simulink model "Sistema_3 (1)"  (R2025b)
settings: Solver=ode23t  StartTime=0.0  StopTime=10.0  RelTol=1e-3
libraries: fl_lib x21, nesl_utility x9, slpidlib x2
settings DataIOCC: ReturnWorkspaceOutputs=off  TimeSaveName=t
settings DebuggingCC: AlgebraicLoopMsg=none  ArtificialAlgebraicLoopMsg=none  MaxConsecutiveZCsMsg=none

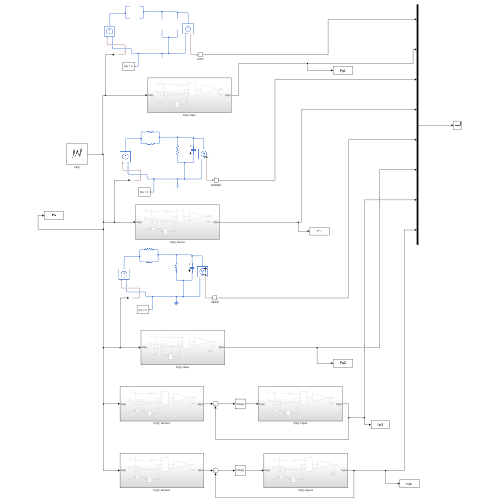
[thumbnail: Simulink's stored preview of the top-level diagram]
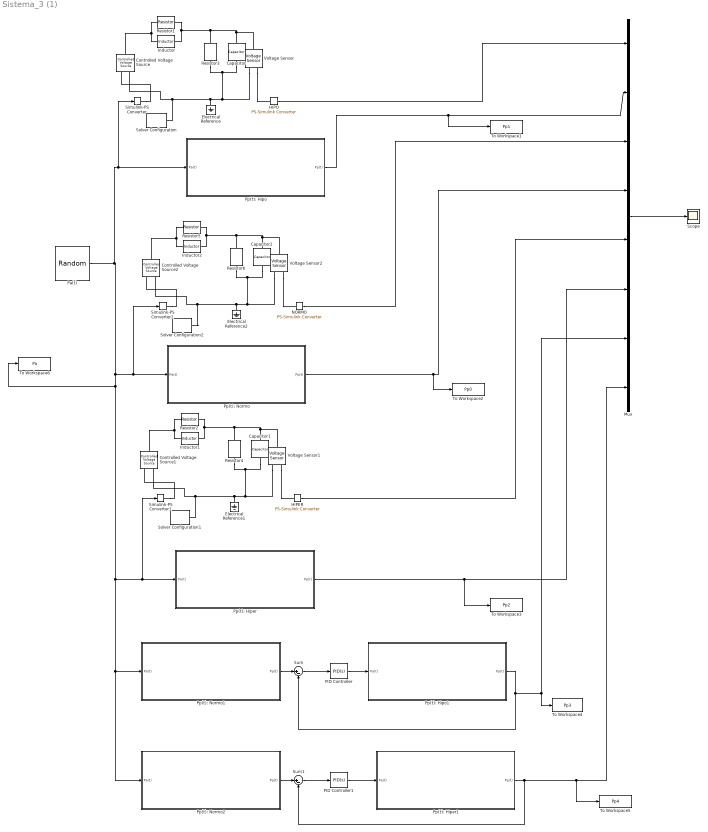
== system Sistema_3 (1) ==
  Capacitor : fl_lib/Electrical/Electrical Elements/Capacitor  c=0.005 F  r=1e-6 Ohm  g=0 1/Ohm  i_specify=off  i_priority=None  i=0 A  i_nominal_specify=off  i_nominal_value=1  i_nominal_unit=A  v_specify=off  v_priority=None  v=0 V  v_nominal_specify=off  v_nominal_value=1  v_nominal_unit=V  vc_specify=off  vc_priority=High  vc=0 V  vc_nominal_specify=off  vc_nominal_value=1  vc_nominal_unit=V
  Capacitor1 : fl_lib/Electrical/Electrical Elements/Capacitor  c=2.500 F  r=1e-6 Ohm  g=0 1/Ohm  i_specify=off  i_priority=None  i=0 A  i_nominal_specify=off  i_nominal_value=1  i_nominal_unit=A  v_specify=off  v_priority=None  v=0 V  v_nominal_specify=off  v_nominal_value=1  v_nominal_unit=V  vc_specify=off  vc_priority=High  vc=0 V  vc_nominal_specify=off  vc_nominal_value=1  vc_nominal_unit=V
  Capacitor2 : fl_lib/Electrical/Electrical Elements/Capacitor  c=1.500 F  r=1e-6 Ohm  g=0 1/Ohm  i_specify=off  i_priority=None  i=0 A  i_nominal_specify=off  i_nominal_value=1  i_nominal_unit=A  v_specify=off  v_priority=None  v=0 V  v_nominal_specify=off  v_nominal_value=1  v_nominal_unit=V  vc_specify=off  vc_priority=High  vc=0 V  vc_nominal_specify=off  vc_nominal_value=1  vc_nominal_unit=V
  Controlled Voltage Source : fl_lib/Electrical/Electrical Sources/Controlled Voltage Source
  Controlled Voltage Source1 : fl_lib/Electrical/Electrical Sources/Controlled Voltage Source
  Controlled Voltage Source2 : fl_lib/Electrical/Electrical Sources/Controlled Voltage Source
  Electrical Reference : fl_lib/Electrical/Electrical Elements/Electrical Reference
  Electrical Reference1 : fl_lib/Electrical/Electrical Elements/Electrical Reference
  Electrical Reference2 : fl_lib/Electrical/Electrical Elements/Electrical Reference
  HIPER : nesl_utility/PS-Simulink Converter  PhysicalDomain=network_engine_domain  SubClassName=ps_output  LeftPortType=input  RightPortType=output  PseudoPeriodic=off  Frequencies=[]  VectorFormat=inherit  Unit=inherit  AffineConversion=off
  HIPO : nesl_utility/PS-Simulink Converter  PhysicalDomain=network_engine_domain  SubClassName=ps_output  LeftPortType=input  RightPortType=output  PseudoPeriodic=off  Frequencies=[]  VectorFormat=inherit  Unit=inherit  AffineConversion=off
  Inductor : fl_lib/Electrical/Electrical Elements/Inductor  l=0.250 H  r=0 Ohm  g=1e-9 1/Ohm  i_specify=off  i_priority=None  i=0 A  i_nominal_specify=off  i_nominal_value=1  i_nominal_unit=A  v_specify=off  v_priority=None  v=0 V  v_nominal_specify=off  v_nominal_value=1  v_nominal_unit=V  i_L_specify=off  i_L_priority=High  i_L=0 A  i_L_nominal_specify=off  i_L_nominal_value=1  i_L_nominal_unit=A
  Inductor1 : fl_lib/Electrical/Electrical Elements/Inductor  l=0.020 H  r=0 Ohm  g=1e-9 1/Ohm  i_specify=off  i_priority=None  i=0 A  i_nominal_specify=off  i_nominal_value=1  i_nominal_unit=A  v_specify=off  v_priority=None  v=0 V  v_nominal_specify=off  v_nominal_value=1  v_nominal_unit=V  i_L_specify=off  i_L_priority=High  i_L=0 A  i_L_nominal_specify=off  i_L_nominal_value=1  i_L_nominal_unit=A
  Inductor2 : fl_lib/Electrical/Electrical Elements/Inductor  l=0.010 H  r=0 Ohm  g=1e-9 1/Ohm  i_specify=off  i_priority=None  i=0 A  i_nominal_specify=off  i_nominal_value=1  i_nominal_unit=A  v_specify=off  v_priority=None  v=0 V  v_nominal_specify=off  v_nominal_value=1  v_nominal_unit=V  i_L_specify=off  i_L_priority=High  i_L=0 A  i_L_nominal_specify=off  i_L_nominal_value=1  i_L_nominal_unit=A
  Mux : Mux  Inputs=8
  NORMO : nesl_utility/PS-Simulink Converter  PhysicalDomain=network_engine_domain  SubClassName=ps_output  LeftPortType=input  RightPortType=output  PseudoPeriodic=off  Frequencies=[]  VectorFormat=inherit  Unit=inherit  AffineConversion=off
  PID Controller : slpidlib/PID Controller  Controller=PID  Form=Parallel  TimeDomain=Continuous-time  UseExternalTs=off  SampleTime=-1  IntegratorMethod=Forward Euler  FilterMethod=Forward Euler  ControllerParametersSource=internal  P=100  I=4003.61190219458  UseKiTs=off  D=0  UseExternalDerivativeSource=off  N=100  UseFilter=on  TunerSelectOption=Transfer Function Based (PID Tuner App)  InitialConditionSource=internal  InitialConditionForIntegrator=0  InitialConditionForFilter=0  DifferentiatorICPrevScaledInput=0  ExternalReset=none  TrackingMode=off  Kt=1  LimitOutput=off  SatLimitsSource=internal  UpperSaturationLimit=inf  LowerSaturationLimit=-inf  LinearizeAsGain=on  AntiWindupMode=none  Kb=1  LimitIntegrator=off  UpperIntegratorSaturationLimit=inf  LowerIntegratorSaturationLimit=-inf  POutMin=[]  POutMax=[]  IOutMin=[]  IOutMax=[]  DOutMin=[]  DOutMax=[]  NOutMin=[]  NOutMax=[]  SumOutMin=[]  SumOutMax=[]  SaturationOutMin=[]  SaturationOutMax=[]  PParamMin=[]  PParamMax=[]  IParamMin=[]  IParamMax=[]  DParamMin=[]  DParamMax=[]  NParamMin=[]  NParamMax=[]  KbParamMin=[]  KbParamMax=[]  KtParamMin=[]  KtParamMax=[]  KbOutMin=[]  KbOutMax=[]  KtOutMin=[]  KtOutMax=[]  IntegratorOutMin=[]  IntegratorOutMax=[]  FilterOutMin=[]  FilterOutMax=[]  SumI1OutMin=[]  SumI1OutMax=[]  SumI2OutMin=[]  SumI2OutMax=[]  SumI3OutMin=[]  SumI3OutMax=[]  SumI4OutMin=[]  SumI4OutMax=[]  SumDOutMin=[]  SumDOutMax=[]  DifferentiatorOutMin=[]  DifferentiatorOutMax=[]  FilterDiffOutCoefMin=[]  FilterDiffOutCoefMax=[]  ReciprocalOutMin=[]  ReciprocalOutMax=[]  SumDenOutMin=[]  SumDenOutMax=[]  SumNumOutMin=[]  SumNumOutMax=[]  DivideOutMin=[]  DivideOutMax=[]  UdiffTsProdOutMin=[]  UdiffTsProdOutMax=[]  NTsProdOutMin=[]  NTsProdOutMax=[]  UintegralTsProdOutMin=[]  UintegralTsProdOutMax=[]  UngainTsProdOutMin=[]  UngainTsProdOutMax=[]  ClampingZeroOutDataTypeStr=Inherit: Inherit via back propagation  ClampingZeroOutMin=[]  ClampingZeroOutMax=[]  FilterDenConstantOutDataTypeStr=Inherit: Inherit via back propagation  FilterDenConstantOutMin=[]  FilterDenConstantOutMax=[]  PCopyOutDataTypeStr=Inherit: Inherit via back propagation  PCopyOutMin=[]  PCopyOutMax=[]  NCopyOutDataTypeStr=Inherit: Inherit via back propagation  NCopyOutMin=[]  NCopyOutMax=[]  IntegratorContinuousStateAttributes=''  IntegratorStateMustResolveToSignalObject=off  IntegratorRTWStateStorageClass=Auto  FilterContinuousStateAttributes=''  FilterStateMustResolveToSignalObject=off  FilterRTWStateStorageClass=Auto  ParallelPVariant=InternalParameters  IdealPVariant=Disabled  IVariant=InternalParameters  DVariant=InternalParameters  IntegratorVariant=Continuous  SatVariant=Disabled  AWVariant=Passthrough  PCopyVariant=Disabled  TRVariant=Disabled  FdbkBlocksVariant=Forward  IdealPFdbkVariant=Disabled  SatFdbkVariant=Disabled  DerivativeFilterVariant=ContFilter  NVariant=InternalParameters  NCopyVariant=Disabled  FilterICVariant=InternalICsFilter  IntegratorICVariant=InternalICs  ExternalResetVariant=Disabled  TRSumVariant=Passthrough  SumFdbkVariant=Disabled  SumVariant=Sum_PID  TsampFilterVariant=InternalTs  TsampNgainVariant=Passthrough  TsampIntegralVariant=Disabled_SignalSpec  ExternalSaturationOutDataTypeStr=Inherit: Same as second input  DerivativeSourceVariant=ErrorSignal  PreIntVariant=InternalPreInt
  PID Controller1 : slpidlib/PID Controller  Controller=PID  Form=Parallel  TimeDomain=Continuous-time  UseExternalTs=off  SampleTime=-1  IntegratorMethod=Forward Euler  FilterMethod=Forward Euler  ControllerParametersSource=internal  P=100  I=4299.5839112344  UseKiTs=off  D=0  UseExternalDerivativeSource=off  N=100  UseFilter=on  TunerSelectOption=Transfer Function Based (PID Tuner App)  InitialConditionSource=internal  InitialConditionForIntegrator=0  InitialConditionForFilter=0  DifferentiatorICPrevScaledInput=0  ExternalReset=none  TrackingMode=off  Kt=1  LimitOutput=off  SatLimitsSource=internal  UpperSaturationLimit=inf  LowerSaturationLimit=-inf  LinearizeAsGain=on  AntiWindupMode=none  Kb=1  LimitIntegrator=off  UpperIntegratorSaturationLimit=inf  LowerIntegratorSaturationLimit=-inf  POutMin=[]  POutMax=[]  IOutMin=[]  IOutMax=[]  DOutMin=[]  DOutMax=[]  NOutMin=[]  NOutMax=[]  SumOutMin=[]  SumOutMax=[]  SaturationOutMin=[]  SaturationOutMax=[]  PParamMin=[]  PParamMax=[]  IParamMin=[]  IParamMax=[]  DParamMin=[]  DParamMax=[]  NParamMin=[]  NParamMax=[]  KbParamMin=[]  KbParamMax=[]  KtParamMin=[]  KtParamMax=[]  KbOutMin=[]  KbOutMax=[]  KtOutMin=[]  KtOutMax=[]  IntegratorOutMin=[]  IntegratorOutMax=[]  FilterOutMin=[]  FilterOutMax=[]  SumI1OutMin=[]  SumI1OutMax=[]  SumI2OutMin=[]  SumI2OutMax=[]  SumI3OutMin=[]  SumI3OutMax=[]  SumI4OutMin=[]  SumI4OutMax=[]  SumDOutMin=[]  SumDOutMax=[]  DifferentiatorOutMin=[]  DifferentiatorOutMax=[]  FilterDiffOutCoefMin=[]  FilterDiffOutCoefMax=[]  ReciprocalOutMin=[]  ReciprocalOutMax=[]  SumDenOutMin=[]  SumDenOutMax=[]  SumNumOutMin=[]  SumNumOutMax=[]  DivideOutMin=[]  DivideOutMax=[]  UdiffTsProdOutMin=[]  UdiffTsProdOutMax=[]  NTsProdOutMin=[]  NTsProdOutMax=[]  UintegralTsProdOutMin=[]  UintegralTsProdOutMax=[]  UngainTsProdOutMin=[]  UngainTsProdOutMax=[]  ClampingZeroOutDataTypeStr=Inherit: Inherit via back propagation  ClampingZeroOutMin=[]  ClampingZeroOutMax=[]  FilterDenConstantOutDataTypeStr=Inherit: Inherit via back propagation  FilterDenConstantOutMin=[]  FilterDenConstantOutMax=[]  PCopyOutDataTypeStr=Inherit: Inherit via back propagation  PCopyOutMin=[]  PCopyOutMax=[]  NCopyOutDataTypeStr=Inherit: Inherit via back propagation  NCopyOutMin=[]  NCopyOutMax=[]  IntegratorContinuousStateAttributes=''  IntegratorStateMustResolveToSignalObject=off  IntegratorRTWStateStorageClass=Auto  FilterContinuousStateAttributes=''  FilterStateMustResolveToSignalObject=off  FilterRTWStateStorageClass=Auto  ParallelPVariant=InternalParameters  IdealPVariant=Disabled  IVariant=InternalParameters  DVariant=InternalParameters  IntegratorVariant=Continuous  SatVariant=Disabled  AWVariant=Passthrough  PCopyVariant=Disabled  TRVariant=Disabled  FdbkBlocksVariant=Forward  IdealPFdbkVariant=Disabled  SatFdbkVariant=Disabled  DerivativeFilterVariant=ContFilter  NVariant=InternalParameters  NCopyVariant=Disabled  FilterICVariant=InternalICsFilter  IntegratorICVariant=InternalICs  ExternalResetVariant=Disabled  TRSumVariant=Passthrough  SumFdbkVariant=Disabled  SumVariant=Sum_PID  TsampFilterVariant=InternalTs  TsampNgainVariant=Passthrough  TsampIntegralVariant=Disabled_SignalSpec  ExternalSaturationOutDataTypeStr=Inherit: Same as second input  DerivativeSourceVariant=ErrorSignal  PreIntVariant=InternalPreInt
  Pa(t) : UniformRandomNumber  Minimum=-0.2  Seed=106  SampleTime=0.5
  Pp(t): Hiper : Subsystem
  Pp(t): Hiper1 : Subsystem
  Pp(t): Hipo : Subsystem
  Pp(t): Hipo1 : Subsystem
  Pp(t): Normo : Subsystem
  Pp(t): Normo1 : Subsystem
  Pp(t): Normo2 : Subsystem
  Resistor1 : fl_lib/Electrical/Electrical Elements/Resistor  R=0.020 Ohm  i_specify=off  i_priority=None  i=0 A  i_nominal_specify=off  i_nominal_value=1  i_nominal_unit=A  v_specify=off  v_priority=None  v=0 V  v_nominal_specify=off  v_nominal_value=1  v_nominal_unit=V
  Resistor2 : fl_lib/Electrical/Electrical Elements/Resistor  R=0.050 Ohm  i_specify=off  i_priority=None  i=0 A  i_nominal_specify=off  i_nominal_value=1  i_nominal_unit=A  v_specify=off  v_priority=None  v=0 V  v_nominal_specify=off  v_nominal_value=1  v_nominal_unit=V
  Resistor3 : fl_lib/Electrical/Electrical Elements/Resistor  R=0.600 Ohm  i_specify=off  i_priority=None  i=0 A  i_nominal_specify=off  i_nominal_value=1  i_nominal_unit=A  v_specify=off  v_priority=None  v=0 V  v_nominal_specify=off  v_nominal_value=1  v_nominal_unit=V
  Resistor4 : fl_lib/Electrical/Electrical Elements/Resistor  R=1.400 Ohm  i_specify=off  i_priority=None  i=0 A  i_nominal_specify=off  i_nominal_value=1  i_nominal_unit=A  v_specify=off  v_priority=None  v=0 V  v_nominal_specify=off  v_nominal_value=1  v_nominal_unit=V
  Resistor5 : fl_lib/Electrical/Electrical Elements/Resistor  R=0.033 Ohm  i_specify=off  i_priority=None  i=0 A  i_nominal_specify=off  i_nominal_value=1  i_nominal_unit=A  v_specify=off  v_priority=None  v=0 V  v_nominal_specify=off  v_nominal_value=1  v_nominal_unit=V
  Resistor6 : fl_lib/Electrical/Electrical Elements/Resistor  R=0.950 Ohm  i_specify=off  i_priority=None  i=0 A  i_nominal_specify=off  i_nominal_value=1  i_nominal_unit=A  v_specify=off  v_priority=None  v=0 V  v_nominal_specify=off  v_nominal_value=1  v_nominal_unit=V
  Scope : Scope
      settings: ActiveDisplayYMinimum=-0.32157829431311108  ActiveDisplayYMaximum=1.2297907338974534
  Simulink-PS Converter : nesl_utility/Simulink-PS Converter  PhysicalDomain=network_engine_domain  SubClassName=ps_input  LeftPortType=input  RightPortType=output  PseudoPeriodic=off  Frequencies=[]  NoiseDistribution=none  NoiseParameters=[]  Unit=1  AffineConversion=off  FilteringAndDerivatives=provide  SimscapeFilterOrder=1  InputFilterTimeConstant=0.001  UdotUserProvided=0
  Simulink-PS Converter1 : nesl_utility/Simulink-PS Converter  PhysicalDomain=network_engine_domain  SubClassName=ps_input  LeftPortType=input  RightPortType=output  PseudoPeriodic=off  Frequencies=[]  NoiseDistribution=none  NoiseParameters=[]  Unit=1  AffineConversion=off  FilteringAndDerivatives=provide  SimscapeFilterOrder=1  InputFilterTimeConstant=0.001  UdotUserProvided=0
  Simulink-PS Converter2 : nesl_utility/Simulink-PS Converter  PhysicalDomain=network_engine_domain  SubClassName=ps_input  LeftPortType=input  RightPortType=output  PseudoPeriodic=off  Frequencies=[]  NoiseDistribution=none  NoiseParameters=[]  Unit=1  AffineConversion=off  FilteringAndDerivatives=provide  SimscapeFilterOrder=1  InputFilterTimeConstant=0.001  UdotUserProvided=0
  Solver Configuration : nesl_utility/Solver Configuration  PhysicalDomain=network_engine_domain  SubClassName=solver  LeftPortType=input  RightPortType=generic  Tones=[]  Harmonics=[]  SimulateNoise=off  Profile=off  UseLocalSampling=off  EnableSwitchedLinearOptims=on  FrequencyDomain=off  UseCCode=off  RelTol=0.001  AbsTol=0.001  MinStep=1e-09  ToWorkspace=off  RevertToSquareIcSolve=off  NumHomotopyIterations=100  PhasorMode=off  PhasorModeNumHarmonics=1  ConsistencySolver=NEWTON_XTOL_AFTER_FTOL  IndexReductionMethod=DerivativeReplacement  DoDC=off  ResidualTolerance=1e-09  ConsistencyTolSource=GLOBAL  ConsistencyAbsTol=0.001  ConsistencyRelTol=0.001  ConsistencyTolFactor=0.001  UseLocalSolver=off  LocalSolverChoice=NE_BACKWARD_EULER_ADVANCER  ResolveIndetEquations=on  FunctionEvalNumThread=1  LocalSolverSampleTime=0.001  DoFixedCost=off  MaxNonlinIter=3  MaxModeIter=2  ComputeImpulses=off  ImpulseIterations=2  LinearAlgebra=auto  LinearAlgebraNumThread=0  EquationFormulation=NE_TIME_EF  DelaysMemoryBudget=1024  AutomaticFiltering=on  FilteringTimeConstant=0.001  PartitionStorageMethod=AS_NEEDED  PartitionMemoryBudget=1024  PartitionMethod=ROBUST  MultibodyUseLocalSolver=off  MultibodyLocalSolverChoice=ODE1  MultibodyLocalSolverSampleTime=0.001
  Solver Configuration1 : nesl_utility/Solver Configuration  PhysicalDomain=network_engine_domain  SubClassName=solver  LeftPortType=input  RightPortType=generic  Tones=[]  Harmonics=[]  SimulateNoise=off  Profile=off  UseLocalSampling=off  EnableSwitchedLinearOptims=on  FrequencyDomain=off  UseCCode=off  RelTol=0.001  AbsTol=0.001  MinStep=1e-09  ToWorkspace=off  RevertToSquareIcSolve=off  NumHomotopyIterations=100  PhasorMode=off  PhasorModeNumHarmonics=1  ConsistencySolver=NEWTON_XTOL_AFTER_FTOL  IndexReductionMethod=DerivativeReplacement  DoDC=off  ResidualTolerance=1e-09  ConsistencyTolSource=GLOBAL  ConsistencyAbsTol=0.001  ConsistencyRelTol=0.001  ConsistencyTolFactor=0.001  UseLocalSolver=off  LocalSolverChoice=NE_BACKWARD_EULER_ADVANCER  ResolveIndetEquations=on  FunctionEvalNumThread=1  LocalSolverSampleTime=0.001  DoFixedCost=off  MaxNonlinIter=3  MaxModeIter=2  ComputeImpulses=off  ImpulseIterations=2  LinearAlgebra=auto  LinearAlgebraNumThread=0  EquationFormulation=NE_TIME_EF  DelaysMemoryBudget=1024  AutomaticFiltering=on  FilteringTimeConstant=0.001  PartitionStorageMethod=AS_NEEDED  PartitionMemoryBudget=1024  PartitionMethod=ROBUST  MultibodyUseLocalSolver=off  MultibodyLocalSolverChoice=ODE1  MultibodyLocalSolverSampleTime=0.001
  Solver Configuration2 : nesl_utility/Solver Configuration  PhysicalDomain=network_engine_domain  SubClassName=solver  LeftPortType=input  RightPortType=generic  Tones=[]  Harmonics=[]  SimulateNoise=off  Profile=off  UseLocalSampling=off  EnableSwitchedLinearOptims=on  FrequencyDomain=off  UseCCode=off  RelTol=0.001  AbsTol=0.001  MinStep=1e-09  ToWorkspace=off  RevertToSquareIcSolve=off  NumHomotopyIterations=100  PhasorMode=off  PhasorModeNumHarmonics=1  ConsistencySolver=NEWTON_XTOL_AFTER_FTOL  IndexReductionMethod=DerivativeReplacement  DoDC=off  ResidualTolerance=1e-09  ConsistencyTolSource=GLOBAL  ConsistencyAbsTol=0.001  ConsistencyRelTol=0.001  ConsistencyTolFactor=0.001  UseLocalSolver=off  LocalSolverChoice=NE_BACKWARD_EULER_ADVANCER  ResolveIndetEquations=on  FunctionEvalNumThread=1  LocalSolverSampleTime=0.001  DoFixedCost=off  MaxNonlinIter=3  MaxModeIter=2  ComputeImpulses=off  ImpulseIterations=2  LinearAlgebra=auto  LinearAlgebraNumThread=0  EquationFormulation=NE_TIME_EF  DelaysMemoryBudget=1024  AutomaticFiltering=on  FilteringTimeConstant=0.001  PartitionStorageMethod=AS_NEEDED  PartitionMemoryBudget=1024  PartitionMethod=ROBUST  MultibodyUseLocalSolver=off  MultibodyLocalSolverChoice=ODE1  MultibodyLocalSolverSampleTime=0.001
  Sum : Sum  Inputs=|+-
  Sum1 : Sum  Inputs=|+-
  To Workspace1 : ToWorkspace  VariableName=Pp1  SampleTime=-1
  To Workspace2 : ToWorkspace  VariableName=Pp0  SampleTime=-1
  To Workspace3 : ToWorkspace  VariableName=Pp2  SampleTime=-1
  To Workspace4 : ToWorkspace  VariableName=Pp3  SampleTime=-1
  To Workspace5 : ToWorkspace  VariableName=Pp4  SampleTime=-1
  To Workspace6 : ToWorkspace  VariableName=Pa  SampleTime=-1
  Voltage Sensor : fl_lib/Electrical/Electrical Sensors/Voltage Sensor
  Voltage Sensor1 : fl_lib/Electrical/Electrical Sensors/Voltage Sensor
  Voltage Sensor2 : fl_lib/Electrical/Electrical Sensors/Voltage Sensor
  wires:
  HIPO/1 -> Mux/1
  Pp(t): Hipo/1(Pp(t)) -> To Workspace1/1, Mux/2
  NORMO/1 -> Mux/3
  HIPER/1 -> Mux/5
  Pp(t): Hiper/1(Pp(t)) -> To Workspace3/1, Mux/6
  Mux/1 -> Scope/1
  Pp(t): Normo/1(Pp(t)) -> To Workspace2/1, Mux/4
  Sum/1 -> PID Controller/1
  Pp(t): Normo1/1(Pp(t)) -> Sum/1
  PID Controller/1 -> Pp(t): Hipo1/1(Pa(t))
  Sum1/1 -> PID Controller1/1
  Pp(t): Normo2/1(Pp(t)) -> Sum1/1
  PID Controller1/1 -> Pp(t): Hiper1/1(Pa(t))
  Pp(t): Hipo1/1(Pp(t)) -> Mux/7, To Workspace4/1, Sum/2
  Pp(t): Hiper1/1(Pp(t)) -> Sum1/2, To Workspace5/1, Mux/8
  Pa(t)/1 -> Pp(t): Hipo/1(Pa(t)), Simulink-PS Converter/1, To Workspace6/1, Pp(t): Normo1/1(Pa(t)), Pp(t): Normo2/1(Pa(t)), Simulink-PS Converter1/1, Pp(t): Hiper/1(Pa(t)), Pp(t): Normo/1(Pa(t)), Simulink-PS Converter2/1
  connections:
  Controlled Voltage Source/RConn2 -- Voltage Sensor/RConn2 -- Capacitor/LConn1 -- Resistor3/RConn1 -- Electrical Reference/LConn1 -- Solver Configuration/RConn1
  Resistor1/RConn1 -- Resistor3/LConn1 -- Voltage Sensor/LConn1 -- Capacitor/RConn1 -- Inductor/LConn1
  Simulink-PS Converter/RConn1 -- Controlled Voltage Source/RConn1
  Voltage Sensor/RConn1 -- HIPO/LConn1
  Resistor1/LConn1 -- Controlled Voltage Source/LConn1 -- Inductor/RConn1
  Resistor2/LConn1 -- Controlled Voltage Source1/LConn1 -- Inductor1/RConn1
  Resistor4/RConn1 -- Capacitor1/LConn1 -- Solver Configuration1/RConn1 -- Controlled Voltage Source1/RConn2 -- Electrical Reference1/LConn1 -- Voltage Sensor1/RConn2
  Resistor2/RConn1 -- Resistor4/LConn1 -- Voltage Sensor1/LConn1 -- Capacitor1/RConn1 -- Inductor1/LConn1
  Simulink-PS Converter1/RConn1 -- Controlled Voltage Source1/RConn1
  Voltage Sensor1/RConn1 -- HIPER/LConn1
  Resistor5/LConn1 -- Controlled Voltage Source2/LConn1 -- Inductor2/RConn1
  Resistor6/RConn1 -- Capacitor2/LConn1 -- Solver Configuration2/RConn1 -- Controlled Voltage Source2/RConn2 -- Electrical Reference2/LConn1 -- Voltage Sensor2/RConn2
  Resistor5/RConn1 -- Resistor6/LConn1 -- Voltage Sensor2/LConn1 -- Capacitor2/RConn1 -- Inductor2/LConn1
  Simulink-PS Converter2/RConn1 -- Controlled Voltage Source2/RConn1
  Voltage Sensor2/RConn1 -- NORMO/LConn1

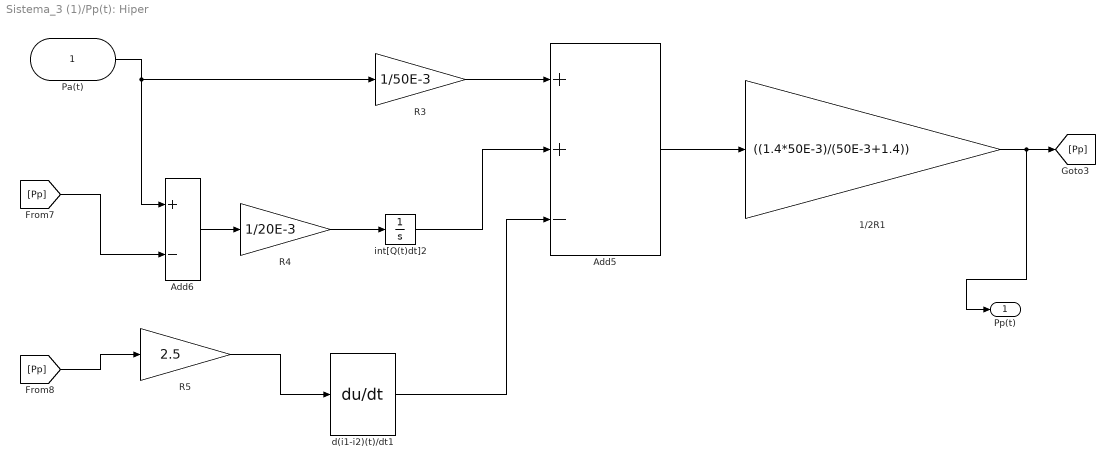
== system Sistema_3 (1)/Pp(t): Hiper ==
  Pa(t) : Inport
  1/2R1 : Gain  Gain=((1.4*50E-3)/(50E-3+1.4))
  Add5 : Sum  Inputs=++-
  Add6 : Sum  Inputs=+-
  R3 : Gain  Gain=1/50E-3
  R4 : Gain  Gain=1/20E-3
  R5 : Gain  Gain=2.5
  d(i1-i2)(t)/dt1 : Derivative
  int[Q(t)dt]2 : Integrator
  Pp(t) : Outport
  wires:
  Pa(t)/1 -> R3/1, Add6/1
  R3/1 -> Add5/1
  [Pp] -> Add6/2
  Add6/1 -> R4/1
  R4/1 -> int[Q(t)dt]2/1
  int[Q(t)dt]2/1 -> Add5/2
  [Pp] -> R5/1
  R5/1 -> d(i1-i2)(t)/dt1/1
  d(i1-i2)(t)/dt1/1 -> Add5/3
  Add5/1 -> 1/2R1/1
  1/2R1/1 -> Pp(t)/1, [Pp]

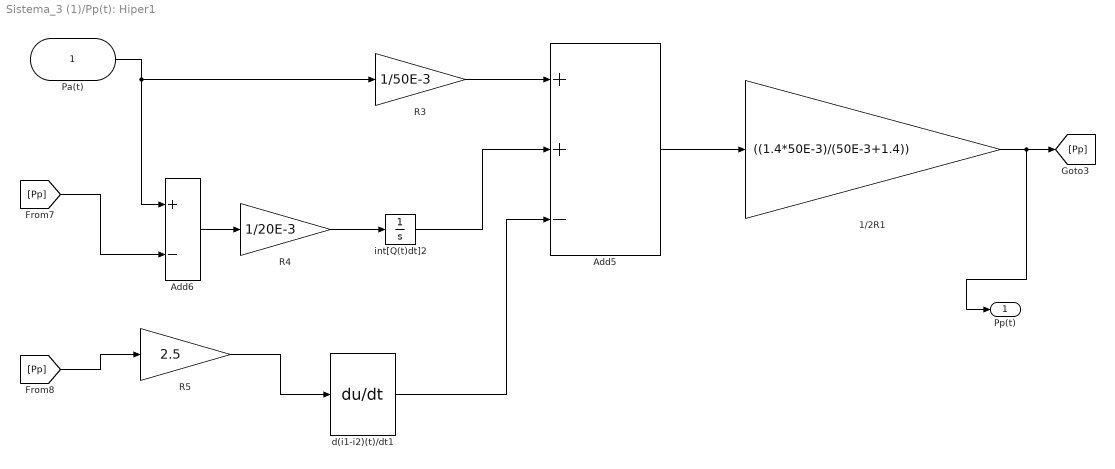
== system Sistema_3 (1)/Pp(t): Hiper1 ==
  Pa(t) : Inport
  1/2R1 : Gain  Gain=((1.4*50E-3)/(50E-3+1.4))
  Add5 : Sum  Inputs=++-
  Add6 : Sum  Inputs=+-
  R3 : Gain  Gain=1/50E-3
  R4 : Gain  Gain=1/20E-3
  R5 : Gain  Gain=2.5
  d(i1-i2)(t)/dt1 : Derivative
  int[Q(t)dt]2 : Integrator
  Pp(t) : Outport
  wires:
  Pa(t)/1 -> R3/1, Add6/1
  R3/1 -> Add5/1
  [Pp] -> Add6/2
  Add6/1 -> R4/1
  R4/1 -> int[Q(t)dt]2/1
  int[Q(t)dt]2/1 -> Add5/2
  [Pp] -> R5/1
  R5/1 -> d(i1-i2)(t)/dt1/1
  d(i1-i2)(t)/dt1/1 -> Add5/3
  Add5/1 -> 1/2R1/1
  1/2R1/1 -> Pp(t)/1, [Pp]

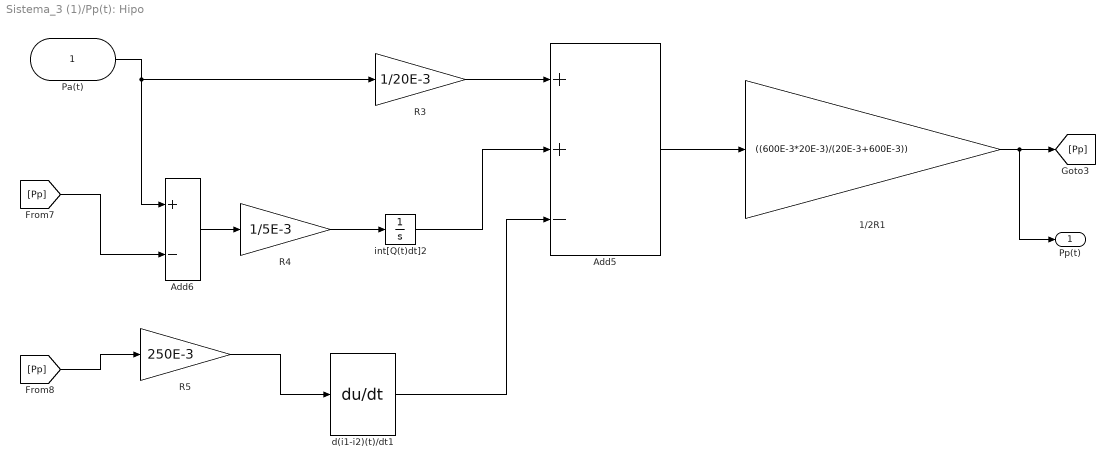
== system Sistema_3 (1)/Pp(t): Hipo ==
  Pa(t) : Inport
  1/2R1 : Gain  Gain=((600E-3*20E-3)/(20E-3+600E-3))
  Add5 : Sum  Inputs=++-
  Add6 : Sum  Inputs=+-
  R3 : Gain  Gain=1/20E-3
  R4 : Gain  Gain=1/5E-3
  R5 : Gain  Gain=250E-3
  d(i1-i2)(t)/dt1 : Derivative
  int[Q(t)dt]2 : Integrator
  Pp(t) : Outport
  wires:
  Pa(t)/1 -> R3/1, Add6/1
  R3/1 -> Add5/1
  [Pp] -> Add6/2
  Add6/1 -> R4/1
  R4/1 -> int[Q(t)dt]2/1
  int[Q(t)dt]2/1 -> Add5/2
  [Pp] -> R5/1
  R5/1 -> d(i1-i2)(t)/dt1/1
  d(i1-i2)(t)/dt1/1 -> Add5/3
  Add5/1 -> 1/2R1/1
  1/2R1/1 -> Pp(t)/1, [Pp]

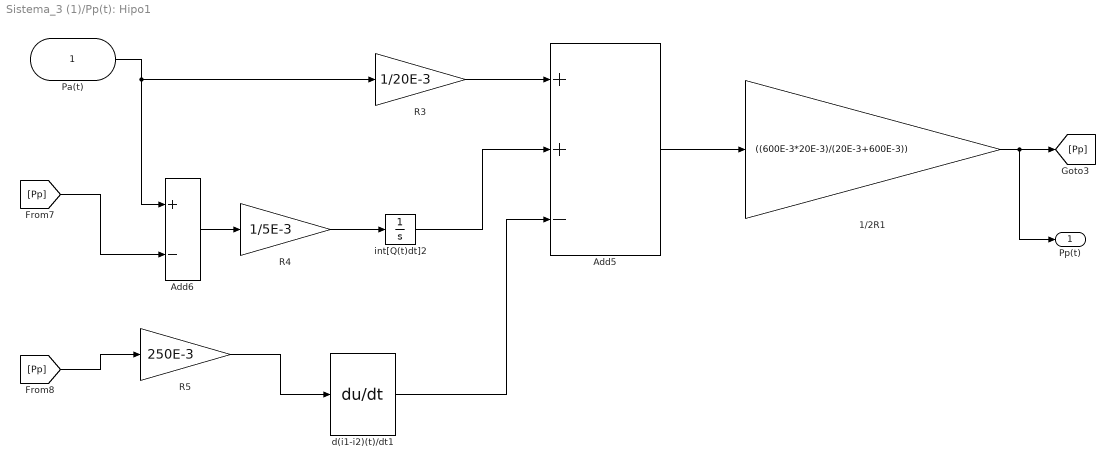
== system Sistema_3 (1)/Pp(t): Hipo1 ==
  Pa(t) : Inport
  1/2R1 : Gain  Gain=((600E-3*20E-3)/(20E-3+600E-3))
  Add5 : Sum  Inputs=++-
  Add6 : Sum  Inputs=+-
  R3 : Gain  Gain=1/20E-3
  R4 : Gain  Gain=1/5E-3
  R5 : Gain  Gain=250E-3
  d(i1-i2)(t)/dt1 : Derivative
  int[Q(t)dt]2 : Integrator
  Pp(t) : Outport
  wires:
  Pa(t)/1 -> R3/1, Add6/1
  R3/1 -> Add5/1
  [Pp] -> Add6/2
  Add6/1 -> R4/1
  R4/1 -> int[Q(t)dt]2/1
  int[Q(t)dt]2/1 -> Add5/2
  [Pp] -> R5/1
  R5/1 -> d(i1-i2)(t)/dt1/1
  d(i1-i2)(t)/dt1/1 -> Add5/3
  Add5/1 -> 1/2R1/1
  1/2R1/1 -> Pp(t)/1, [Pp]

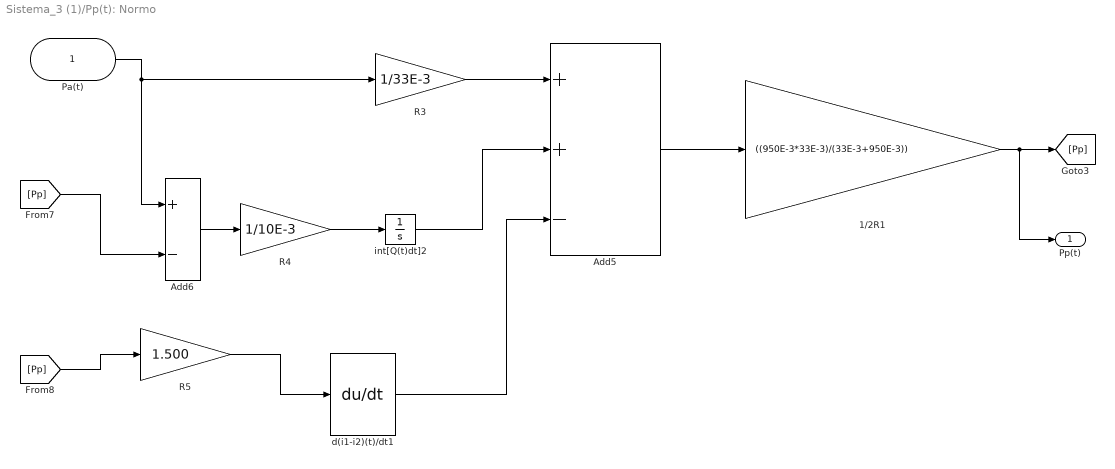
== system Sistema_3 (1)/Pp(t): Normo ==
  Pa(t) : Inport
  1/2R1 : Gain  Gain=((950E-3*33E-3)/(33E-3+950E-3))
  Add5 : Sum  Inputs=++-
  Add6 : Sum  Inputs=+-
  R3 : Gain  Gain=1/33E-3
  R4 : Gain  Gain=1/10E-3
  R5 : Gain  Gain=1.500
  d(i1-i2)(t)/dt1 : Derivative
  int[Q(t)dt]2 : Integrator
  Pp(t) : Outport
  wires:
  Pa(t)/1 -> R3/1, Add6/1
  R3/1 -> Add5/1
  [Pp] -> Add6/2
  Add6/1 -> R4/1
  R4/1 -> int[Q(t)dt]2/1
  int[Q(t)dt]2/1 -> Add5/2
  [Pp] -> R5/1
  R5/1 -> d(i1-i2)(t)/dt1/1
  d(i1-i2)(t)/dt1/1 -> Add5/3
  Add5/1 -> 1/2R1/1
  1/2R1/1 -> Pp(t)/1, [Pp]

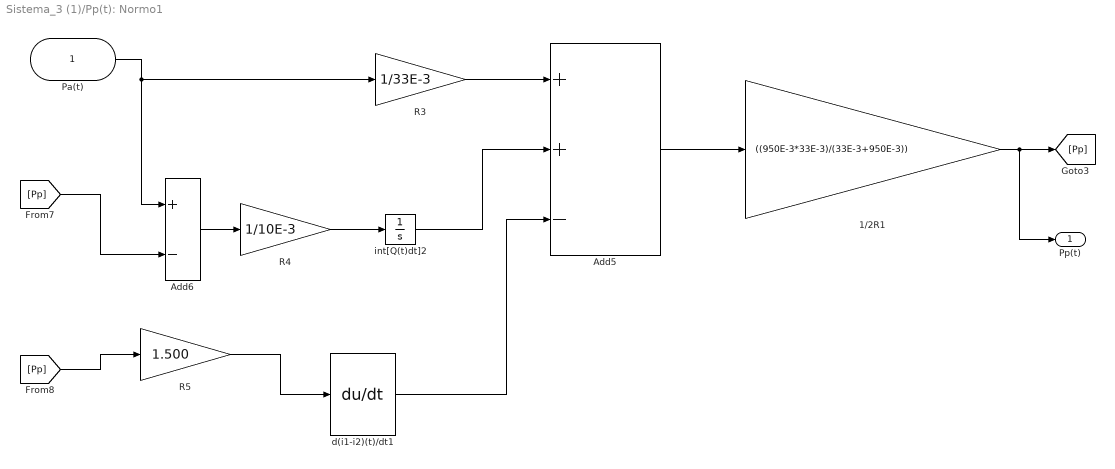
== system Sistema_3 (1)/Pp(t): Normo1 ==
  Pa(t) : Inport
  1/2R1 : Gain  Gain=((950E-3*33E-3)/(33E-3+950E-3))
  Add5 : Sum  Inputs=++-
  Add6 : Sum  Inputs=+-
  R3 : Gain  Gain=1/33E-3
  R4 : Gain  Gain=1/10E-3
  R5 : Gain  Gain=1.500
  d(i1-i2)(t)/dt1 : Derivative
  int[Q(t)dt]2 : Integrator
  Pp(t) : Outport
  wires:
  Pa(t)/1 -> R3/1, Add6/1
  R3/1 -> Add5/1
  [Pp] -> Add6/2
  Add6/1 -> R4/1
  R4/1 -> int[Q(t)dt]2/1
  int[Q(t)dt]2/1 -> Add5/2
  [Pp] -> R5/1
  R5/1 -> d(i1-i2)(t)/dt1/1
  d(i1-i2)(t)/dt1/1 -> Add5/3
  Add5/1 -> 1/2R1/1
  1/2R1/1 -> Pp(t)/1, [Pp]

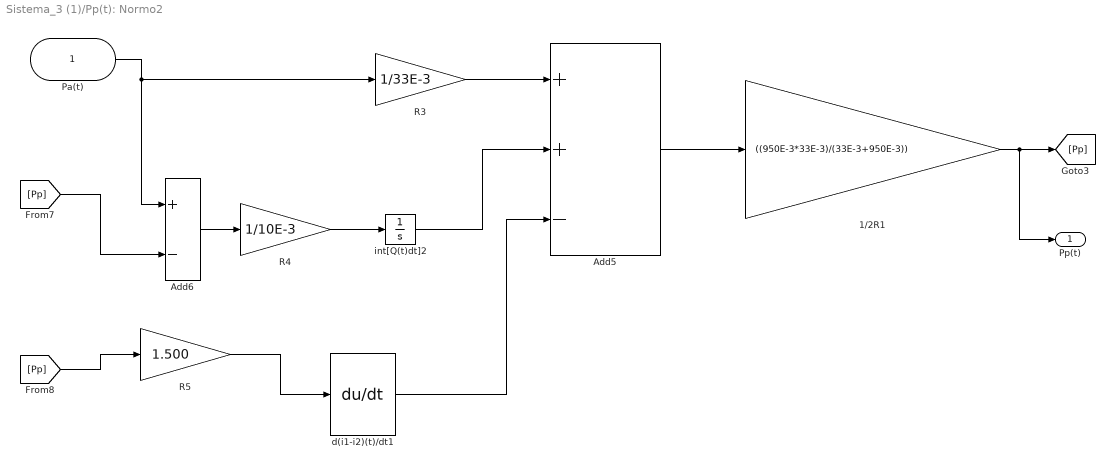
== system Sistema_3 (1)/Pp(t): Normo2 ==
  Pa(t) : Inport
  1/2R1 : Gain  Gain=((950E-3*33E-3)/(33E-3+950E-3))
  Add5 : Sum  Inputs=++-
  Add6 : Sum  Inputs=+-
  R3 : Gain  Gain=1/33E-3
  R4 : Gain  Gain=1/10E-3
  R5 : Gain  Gain=1.500
  d(i1-i2)(t)/dt1 : Derivative
  int[Q(t)dt]2 : Integrator
  Pp(t) : Outport
  wires:
  Pa(t)/1 -> R3/1, Add6/1
  R3/1 -> Add5/1
  [Pp] -> Add6/2
  Add6/1 -> R4/1
  R4/1 -> int[Q(t)dt]2/1
  int[Q(t)dt]2/1 -> Add5/2
  [Pp] -> R5/1
  R5/1 -> d(i1-i2)(t)/dt1/1
  d(i1-i2)(t)/dt1/1 -> Add5/3
  Add5/1 -> 1/2R1/1
  1/2R1/1 -> Pp(t)/1, [Pp]
